simulink model "modelo"  (Simulink 7.7)
settings: Solver=ode45  StartTime=0.0  StopTime=10.0  RelTol=1e-3
settings Model: Creator=Guillermo  LastModifiedBy=Guillermo
settings OptimizationCC: InlineInvariantSignals=on  InitFltsAndDblsToZero=on
settings DebuggingCC: SaveWithParameterizedLinksMsg=none  SignalResolutionControl=TryResolveAllWithWarning  MultiTaskDSMMsg=warning  MultiTaskCondExecSysMsg=none  StrictBusMsg=None
settings RTWCC: IncludeERTFirstTime=on
settings GRTTargetCC: TargetFcnLib=ansi_tfl_tmw.mat

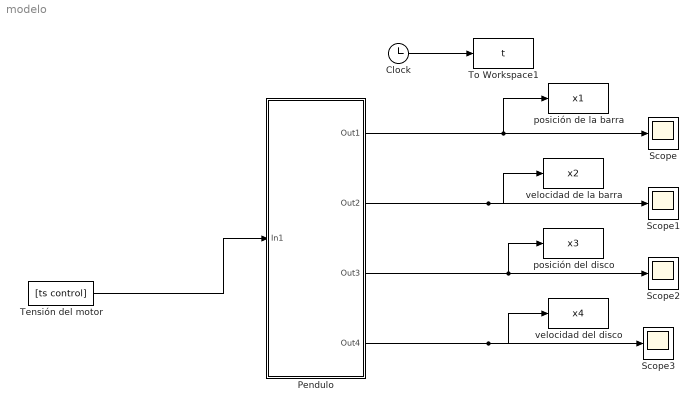
== system modelo ==
  Clock : Clock
      settings: Decimation=10
  Pendulo : Subsystem
  Scope{,1..3} (4 alike) : Scope
      Scope2 settings: SaveName=ScopeData2
      Scope3 settings: SaveName=ScopeData3
  Tensión del motor : FromWorkspace  VariableName=[ts control]  SampleTime=0.01
  To Workspace1 : ToWorkspace  VariableName=t  SampleTime=-1  SaveFormat=Array
  posición de la barra : ToWorkspace  VariableName=x1  SampleTime=-1  SaveFormat=Array
  posición del disco : ToWorkspace  VariableName=x3  SampleTime=-1  SaveFormat=Array
  velocidad de la barra : ToWorkspace  VariableName=x2  SampleTime=-1  SaveFormat=Array
  velocidad del disco : ToWorkspace  VariableName=x4  SampleTime=-1  SaveFormat=Array
  wires:
  Clock/1 -> To Workspace1/1
  Pendulo/1(Out1) -> Scope/1, posición de la barra/1
  Pendulo/2(Out2) -> velocidad de la barra/1, Scope1/1
  Pendulo/3(Out3) -> posición del disco/1, Scope2/1
  Pendulo/4(Out4) -> velocidad del disco/1, Scope3/1
  Tensión del motor/1 -> Pendulo/1(In1)

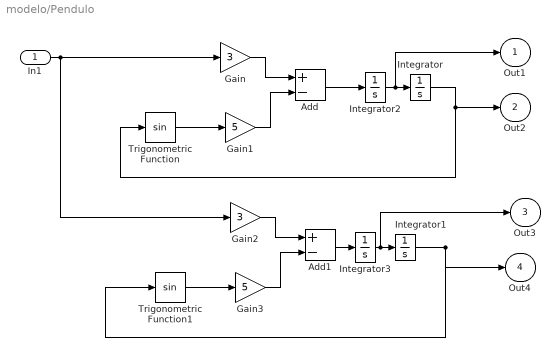
== system modelo/Pendulo ==
  In1 : Inport
  Add : Sum  Inputs=+-
  Add1 : Sum  Inputs=+-
  Gain : Gain  Gain=3
  Gain1 : Gain  Gain=5
  Gain2 : Gain  Gain=3
  Gain3 : Gain  Gain=5
  Integrator{,1..3} (4 alike) : Integrator
  Trigonometric Function : Trigonometry
  Trigonometric Function1 : Trigonometry
  Out1 : Outport
  Out2 : Outport  Port=2
  Out3 : Outport  Port=3
  Out4 : Outport  Port=4
  wires:
  Trigonometric Function/1 -> Gain1/1
  Gain1/1 -> Add/2
  Add/1 -> Integrator2/1
  Gain/1 -> Add/1
  In1/1 -> Gain/1, Gain2/1
  Trigonometric Function1/1 -> Gain3/1
  Gain3/1 -> Add1/2
  Add1/1 -> Integrator3/1
  Gain2/1 -> Add1/1
  Integrator1/1 -> Trigonometric Function1/1, Out4/1
  Integrator/1 -> Trigonometric Function/1, Out2/1
  Integrator2/1 -> Integrator/1, Out1/1
  Integrator3/1 -> Integrator1/1, Out3/1
